simulink model "untitled"  (R2014a)
settings: Solver=ode4  StartTime=0.0  StopTime=4  FixedStep=0.003  RelTol=1e-3
libraries: slrtlib x2, xpcnilib x2
settings Model: SimulationMode=external  BufferReuse=off  Creator=Lab322  LastModifiedBy=Lab322
settings SolverCC: EnableConcurrentExecution=on
settings OptimizationCC: BlockReduction=off  OptimizeBlockIOStorage=off  BufferReuse=off  GlobalBufferReuse=off  ExpressionFolding=off  LocalBlockOutputs=off
settings HardwareCC: ProdIntDivRoundTo=Zero  ProdEndianess=LittleEndian  ProdHWDeviceType=Generic->32-bit x86 compatible
settings RTWCC: SystemTargetFile=slrt.tlc  TemplateMakefile=slrt_default_tmf  Description=Simulink Real-Time  ProcessScript=slrt_make_rtw_hook  RTWCompilerOptimization=On
settings SimulinkRealTimeCC: GeneratePreprocessorConditionals=Disable all  EnableShiftOperators=on

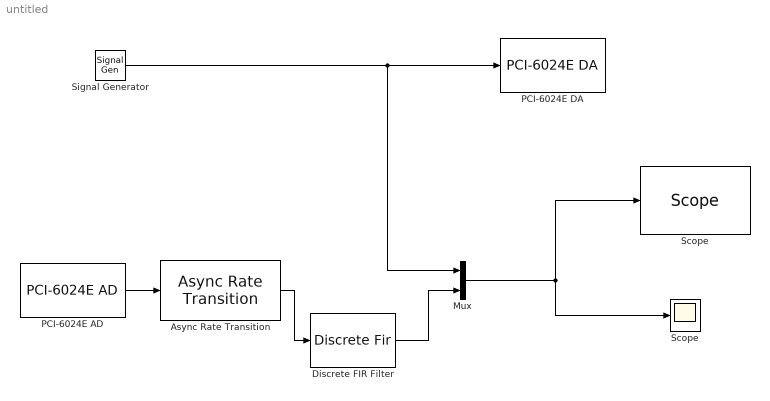
== system untitled ==
  "Async Rate Transition " : slrtlib/Asynchronous Event/Async Rate Transition   sample_time=0.003
  Discrete FIR Filter : DiscreteFir  InputProcessing=Columns as channels (frame based)
  Mux : Mux  Inputs=2
  PCI-6024E AD : xpcnilib/A//D/E Series/PCI-6024E AD  channel=[9]  range=[-10]  coupling=[0]  sampletime=0.006  slot=-1
  PCI-6024E DA : xpcnilib/D//A/E Series/PCI-6024E DA  channel=[1]  reset=[1]  initValue=[0]  sampletime=-1  slot=-1
  Scope : Scope
  "Scope " : slrtlib/Displays and Logging/Scope   scopeno=1  scopetype=Target  autostart=on  viewmode=Graphical redraw  formatstr='%15.6f'  grid=on  ylimits=[0,0]  nosamples=600  noprepostsamples=0  interleave=1  triggermode=FreeRun  triggersignal=1  trigsignalfromport=off  triggerlevel=0.0  triggerslope=Either  triggerscope=1  triggersample=0  filename=data.dat  mode=Lazy  writesize=512  autorestart=off  dynamicfilemode=off  maxwritefilesize=512*1024^2
  Signal Generator : SignalGenerator  Amplitude=4  Frequency=5
  wires:
  Signal Generator/1 -> Mux/1, PCI-6024E DA/1
  Mux/1 -> "Scope "/1, Scope/1
  Discrete FIR Filter/1 -> Mux/2
  "Async Rate Transition "/1 -> Discrete FIR Filter/1
  PCI-6024E AD/1 -> "Async Rate Transition "/1
